simulink model "Y_Model_20_Loads"  (R2018b)
settings: Solver=VariableStepAuto  StartTime=0.0  StopTime=sim_t  RelTol=1e-3
values from neighbouring files (symbols this model uses):
  dt = 5e-5    (= 5e-05)    [Y_multi_sim_loads.m]
  L = ones(num_sims, num_loads) * L_max    [Y_multi_sim_loads.m]
  P = rand(num_sims, num_loads) * (P_max - P_min) + P_min    [Y_multi_sim_loads.m]
  R = ones(num_sims, num_loads) * R_max    [Y_multi_sim_loads.m]
libraries: powerlib x270, powerlib_meascontrol x56
(part 3 of 4)

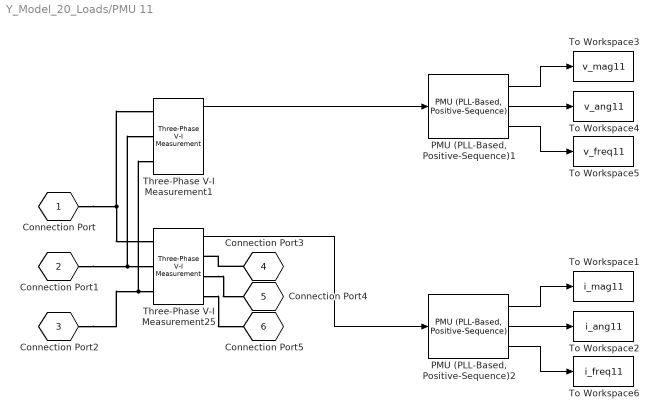
== system Y_Model_20_Loads/PMU 11 ==
  "PMU (PLL-Based, Positive-Sequence)1" : powerlib_meascontrol/Measurements/PMU (PLL-Based, Positive-Sequence)  nominalFrequency=50  samplingRate=64  reportingFactor=64
      settings: SourceProductName=Simscape Electrical  SourceProductBaseCode=PS
  "PMU (PLL-Based, Positive-Sequence)2" : powerlib_meascontrol/Measurements/PMU (PLL-Based, Positive-Sequence)  nominalFrequency=50  samplingRate=64  reportingFactor=64
      settings: SourceProductName=Simscape Electrical  SourceProductBaseCode=PS
  Three-Phase V-I Measurement1 : powerlib/Measurements/Three-Phase V-I Measurement  VoltageMeasurement=phase-to-ground  SetLabelV=off  LabelV=Vabc  Vpu=off  VpuLL=off  CurrentMeasurement=no  SetLabelI=off  LabelI=Iabc  Ipu=off  Pbase=100e6  Vbase=500e3  OutputType=Complex  PhasorSimulation=off  PSBequivalent=0
      settings: SourceProductName=Simscape Electrical
  Three-Phase V-I Measurement25 : powerlib/Measurements/Three-Phase V-I Measurement  VoltageMeasurement=no  SetLabelV=off  LabelV=Vabc  Vpu=off  VpuLL=off  CurrentMeasurement=yes  SetLabelI=off  LabelI=Iabc  Ipu=off  Pbase=100e6  Vbase=500e3  OutputType=Complex  PhasorSimulation=off  PSBequivalent=0
      settings: SourceProductName=Simscape Electrical
  To Workspace1 : ToWorkspace  VariableName=i_mag11  SampleTime=-1
  To Workspace2 : ToWorkspace  VariableName=i_ang11  SampleTime=-1
  To Workspace3 : ToWorkspace  VariableName=v_mag11  SampleTime=-1
  To Workspace4 : ToWorkspace  VariableName=v_ang11  SampleTime=-1
  To Workspace5 : ToWorkspace  VariableName=v_freq11  SampleTime=-1
  To Workspace6 : ToWorkspace  VariableName=i_freq11  SampleTime=-1
  Connection Port : PMIOPort  Tag=PMCPort  Side=Left
  Connection Port1 : PMIOPort  Tag=PMCPort  Port=2  Side=Left
  Connection Port2 : PMIOPort  Tag=PMCPort  Port=3  Side=Left
  Connection Port3 : PMIOPort  Tag=PMCPort  Port=4  Side=Right
  Connection Port4 : PMIOPort  Tag=PMCPort  Port=5  Side=Right
  Connection Port5 : PMIOPort  Tag=PMCPort  Port=6  Side=Right
  wires:
  "PMU (PLL-Based, Positive-Sequence)1"/3 -> To Workspace5/1
  "PMU (PLL-Based, Positive-Sequence)1"/2 -> To Workspace4/1
  "PMU (PLL-Based, Positive-Sequence)1"/1 -> To Workspace3/1
  "PMU (PLL-Based, Positive-Sequence)2"/3 -> To Workspace6/1
  "PMU (PLL-Based, Positive-Sequence)2"/1 -> To Workspace1/1
  "PMU (PLL-Based, Positive-Sequence)2"/2 -> To Workspace2/1
  Three-Phase V-I Measurement25/1 -> "PMU (PLL-Based, Positive-Sequence)2"/1
  Three-Phase V-I Measurement1/1 -> "PMU (PLL-Based, Positive-Sequence)1"/1
  connections:
  Three-Phase V-I Measurement25/LConn1 -- Connection Port/RConn1 -- Three-Phase V-I Measurement1/LConn1
  Connection Port1/RConn1 -- Three-Phase V-I Measurement1/LConn2 -- Three-Phase V-I Measurement25/LConn2
  Connection Port2/RConn1 -- Three-Phase V-I Measurement25/LConn3 -- Three-Phase V-I Measurement1/LConn3
  Connection Port3/RConn1 -- Three-Phase V-I Measurement25/RConn1
  Three-Phase V-I Measurement25/RConn2 -- Connection Port4/RConn1
  Three-Phase V-I Measurement25/RConn3 -- Connection Port5/RConn1

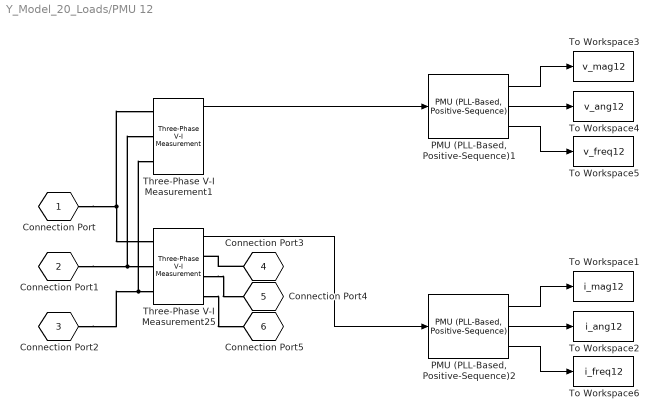
== system Y_Model_20_Loads/PMU 12 ==
  "PMU (PLL-Based, Positive-Sequence)1" : powerlib_meascontrol/Measurements/PMU (PLL-Based, Positive-Sequence)  nominalFrequency=50  samplingRate=64  reportingFactor=64
      settings: SourceProductName=Simscape Electrical  SourceProductBaseCode=PS
  "PMU (PLL-Based, Positive-Sequence)2" : powerlib_meascontrol/Measurements/PMU (PLL-Based, Positive-Sequence)  nominalFrequency=50  samplingRate=64  reportingFactor=64
      settings: SourceProductName=Simscape Electrical  SourceProductBaseCode=PS
  Three-Phase V-I Measurement1 : powerlib/Measurements/Three-Phase V-I Measurement  VoltageMeasurement=phase-to-ground  SetLabelV=off  LabelV=Vabc  Vpu=off  VpuLL=off  CurrentMeasurement=no  SetLabelI=off  LabelI=Iabc  Ipu=off  Pbase=100e6  Vbase=500e3  OutputType=Complex  PhasorSimulation=off  PSBequivalent=0
      settings: SourceProductName=Simscape Electrical
  Three-Phase V-I Measurement25 : powerlib/Measurements/Three-Phase V-I Measurement  VoltageMeasurement=no  SetLabelV=off  LabelV=Vabc  Vpu=off  VpuLL=off  CurrentMeasurement=yes  SetLabelI=off  LabelI=Iabc  Ipu=off  Pbase=100e6  Vbase=500e3  OutputType=Complex  PhasorSimulation=off  PSBequivalent=0
      settings: SourceProductName=Simscape Electrical
  To Workspace1 : ToWorkspace  VariableName=i_mag12  SampleTime=-1
  To Workspace2 : ToWorkspace  VariableName=i_ang12  SampleTime=-1
  To Workspace3 : ToWorkspace  VariableName=v_mag12  SampleTime=-1
  To Workspace4 : ToWorkspace  VariableName=v_ang12  SampleTime=-1
  To Workspace5 : ToWorkspace  VariableName=v_freq12  SampleTime=-1
  To Workspace6 : ToWorkspace  VariableName=i_freq12  SampleTime=-1
  Connection Port : PMIOPort  Tag=PMCPort  Side=Left
  Connection Port1 : PMIOPort  Tag=PMCPort  Port=2  Side=Left
  Connection Port2 : PMIOPort  Tag=PMCPort  Port=3  Side=Left
  Connection Port3 : PMIOPort  Tag=PMCPort  Port=4  Side=Right
  Connection Port4 : PMIOPort  Tag=PMCPort  Port=5  Side=Right
  Connection Port5 : PMIOPort  Tag=PMCPort  Port=6  Side=Right
  wires:
  "PMU (PLL-Based, Positive-Sequence)1"/3 -> To Workspace5/1
  "PMU (PLL-Based, Positive-Sequence)1"/2 -> To Workspace4/1
  "PMU (PLL-Based, Positive-Sequence)1"/1 -> To Workspace3/1
  "PMU (PLL-Based, Positive-Sequence)2"/3 -> To Workspace6/1
  "PMU (PLL-Based, Positive-Sequence)2"/1 -> To Workspace1/1
  "PMU (PLL-Based, Positive-Sequence)2"/2 -> To Workspace2/1
  Three-Phase V-I Measurement25/1 -> "PMU (PLL-Based, Positive-Sequence)2"/1
  Three-Phase V-I Measurement1/1 -> "PMU (PLL-Based, Positive-Sequence)1"/1
  connections:
  Three-Phase V-I Measurement25/LConn1 -- Connection Port/RConn1 -- Three-Phase V-I Measurement1/LConn1
  Connection Port1/RConn1 -- Three-Phase V-I Measurement1/LConn2 -- Three-Phase V-I Measurement25/LConn2
  Connection Port2/RConn1 -- Three-Phase V-I Measurement25/LConn3 -- Three-Phase V-I Measurement1/LConn3
  Connection Port3/RConn1 -- Three-Phase V-I Measurement25/RConn1
  Three-Phase V-I Measurement25/RConn2 -- Connection Port4/RConn1
  Three-Phase V-I Measurement25/RConn3 -- Connection Port5/RConn1

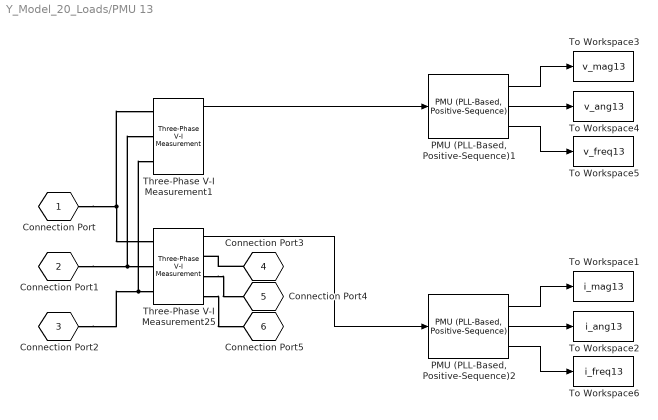
== system Y_Model_20_Loads/PMU 13 ==
  "PMU (PLL-Based, Positive-Sequence)1" : powerlib_meascontrol/Measurements/PMU (PLL-Based, Positive-Sequence)  nominalFrequency=50  samplingRate=64  reportingFactor=64
      settings: SourceProductName=Simscape Electrical  SourceProductBaseCode=PS
  "PMU (PLL-Based, Positive-Sequence)2" : powerlib_meascontrol/Measurements/PMU (PLL-Based, Positive-Sequence)  nominalFrequency=50  samplingRate=64  reportingFactor=64
      settings: SourceProductName=Simscape Electrical  SourceProductBaseCode=PS
  Three-Phase V-I Measurement1 : powerlib/Measurements/Three-Phase V-I Measurement  VoltageMeasurement=phase-to-ground  SetLabelV=off  LabelV=Vabc  Vpu=off  VpuLL=off  CurrentMeasurement=no  SetLabelI=off  LabelI=Iabc  Ipu=off  Pbase=100e6  Vbase=500e3  OutputType=Complex  PhasorSimulation=off  PSBequivalent=0
      settings: SourceProductName=Simscape Electrical
  Three-Phase V-I Measurement25 : powerlib/Measurements/Three-Phase V-I Measurement  VoltageMeasurement=no  SetLabelV=off  LabelV=Vabc  Vpu=off  VpuLL=off  CurrentMeasurement=yes  SetLabelI=off  LabelI=Iabc  Ipu=off  Pbase=100e6  Vbase=500e3  OutputType=Complex  PhasorSimulation=off  PSBequivalent=0
      settings: SourceProductName=Simscape Electrical
  To Workspace1 : ToWorkspace  VariableName=i_mag13  SampleTime=-1
  To Workspace2 : ToWorkspace  VariableName=i_ang13  SampleTime=-1
  To Workspace3 : ToWorkspace  VariableName=v_mag13  SampleTime=-1
  To Workspace4 : ToWorkspace  VariableName=v_ang13  SampleTime=-1
  To Workspace5 : ToWorkspace  VariableName=v_freq13  SampleTime=-1
  To Workspace6 : ToWorkspace  VariableName=i_freq13  SampleTime=-1
  Connection Port : PMIOPort  Tag=PMCPort  Side=Left
  Connection Port1 : PMIOPort  Tag=PMCPort  Port=2  Side=Left
  Connection Port2 : PMIOPort  Tag=PMCPort  Port=3  Side=Left
  Connection Port3 : PMIOPort  Tag=PMCPort  Port=4  Side=Right
  Connection Port4 : PMIOPort  Tag=PMCPort  Port=5  Side=Right
  Connection Port5 : PMIOPort  Tag=PMCPort  Port=6  Side=Right
  wires:
  "PMU (PLL-Based, Positive-Sequence)1"/3 -> To Workspace5/1
  "PMU (PLL-Based, Positive-Sequence)1"/2 -> To Workspace4/1
  "PMU (PLL-Based, Positive-Sequence)1"/1 -> To Workspace3/1
  "PMU (PLL-Based, Positive-Sequence)2"/3 -> To Workspace6/1
  "PMU (PLL-Based, Positive-Sequence)2"/1 -> To Workspace1/1
  "PMU (PLL-Based, Positive-Sequence)2"/2 -> To Workspace2/1
  Three-Phase V-I Measurement25/1 -> "PMU (PLL-Based, Positive-Sequence)2"/1
  Three-Phase V-I Measurement1/1 -> "PMU (PLL-Based, Positive-Sequence)1"/1
  connections:
  Three-Phase V-I Measurement25/LConn1 -- Connection Port/RConn1 -- Three-Phase V-I Measurement1/LConn1
  Connection Port1/RConn1 -- Three-Phase V-I Measurement1/LConn2 -- Three-Phase V-I Measurement25/LConn2
  Connection Port2/RConn1 -- Three-Phase V-I Measurement25/LConn3 -- Three-Phase V-I Measurement1/LConn3
  Connection Port3/RConn1 -- Three-Phase V-I Measurement25/RConn1
  Three-Phase V-I Measurement25/RConn2 -- Connection Port4/RConn1
  Three-Phase V-I Measurement25/RConn3 -- Connection Port5/RConn1

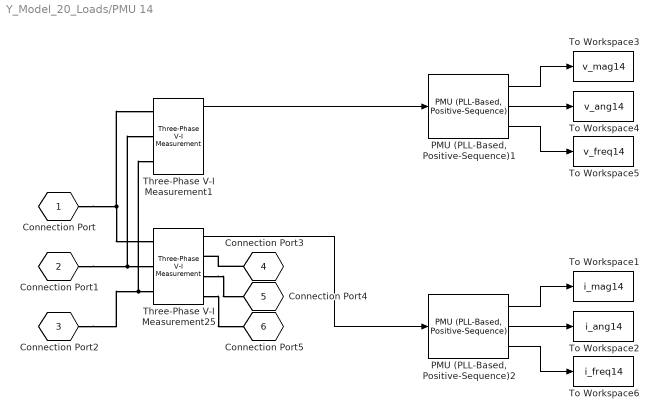
== system Y_Model_20_Loads/PMU 14 ==
  "PMU (PLL-Based, Positive-Sequence)1" : powerlib_meascontrol/Measurements/PMU (PLL-Based, Positive-Sequence)  nominalFrequency=50  samplingRate=64  reportingFactor=64
      settings: SourceProductName=Simscape Electrical  SourceProductBaseCode=PS
  "PMU (PLL-Based, Positive-Sequence)2" : powerlib_meascontrol/Measurements/PMU (PLL-Based, Positive-Sequence)  nominalFrequency=50  samplingRate=64  reportingFactor=64
      settings: SourceProductName=Simscape Electrical  SourceProductBaseCode=PS
  Three-Phase V-I Measurement1 : powerlib/Measurements/Three-Phase V-I Measurement  VoltageMeasurement=phase-to-ground  SetLabelV=off  LabelV=Vabc  Vpu=off  VpuLL=off  CurrentMeasurement=no  SetLabelI=off  LabelI=Iabc  Ipu=off  Pbase=100e6  Vbase=500e3  OutputType=Complex  PhasorSimulation=off  PSBequivalent=0
      settings: SourceProductName=Simscape Electrical
  Three-Phase V-I Measurement25 : powerlib/Measurements/Three-Phase V-I Measurement  VoltageMeasurement=no  SetLabelV=off  LabelV=Vabc  Vpu=off  VpuLL=off  CurrentMeasurement=yes  SetLabelI=off  LabelI=Iabc  Ipu=off  Pbase=100e6  Vbase=500e3  OutputType=Complex  PhasorSimulation=off  PSBequivalent=0
      settings: SourceProductName=Simscape Electrical
  To Workspace1 : ToWorkspace  VariableName=i_mag14  SampleTime=-1
  To Workspace2 : ToWorkspace  VariableName=i_ang14  SampleTime=-1
  To Workspace3 : ToWorkspace  VariableName=v_mag14  SampleTime=-1
  To Workspace4 : ToWorkspace  VariableName=v_ang14  SampleTime=-1
  To Workspace5 : ToWorkspace  VariableName=v_freq14  SampleTime=-1
  To Workspace6 : ToWorkspace  VariableName=i_freq14  SampleTime=-1
  Connection Port : PMIOPort  Tag=PMCPort  Side=Left
  Connection Port1 : PMIOPort  Tag=PMCPort  Port=2  Side=Left
  Connection Port2 : PMIOPort  Tag=PMCPort  Port=3  Side=Left
  Connection Port3 : PMIOPort  Tag=PMCPort  Port=4  Side=Right
  Connection Port4 : PMIOPort  Tag=PMCPort  Port=5  Side=Right
  Connection Port5 : PMIOPort  Tag=PMCPort  Port=6  Side=Right
  wires:
  "PMU (PLL-Based, Positive-Sequence)1"/3 -> To Workspace5/1
  "PMU (PLL-Based, Positive-Sequence)1"/2 -> To Workspace4/1
  "PMU (PLL-Based, Positive-Sequence)1"/1 -> To Workspace3/1
  "PMU (PLL-Based, Positive-Sequence)2"/3 -> To Workspace6/1
  "PMU (PLL-Based, Positive-Sequence)2"/1 -> To Workspace1/1
  "PMU (PLL-Based, Positive-Sequence)2"/2 -> To Workspace2/1
  Three-Phase V-I Measurement25/1 -> "PMU (PLL-Based, Positive-Sequence)2"/1
  Three-Phase V-I Measurement1/1 -> "PMU (PLL-Based, Positive-Sequence)1"/1
  connections:
  Three-Phase V-I Measurement25/LConn1 -- Connection Port/RConn1 -- Three-Phase V-I Measurement1/LConn1
  Connection Port1/RConn1 -- Three-Phase V-I Measurement1/LConn2 -- Three-Phase V-I Measurement25/LConn2
  Connection Port2/RConn1 -- Three-Phase V-I Measurement25/LConn3 -- Three-Phase V-I Measurement1/LConn3
  Connection Port3/RConn1 -- Three-Phase V-I Measurement25/RConn1
  Three-Phase V-I Measurement25/RConn2 -- Connection Port4/RConn1
  Three-Phase V-I Measurement25/RConn3 -- Connection Port5/RConn1

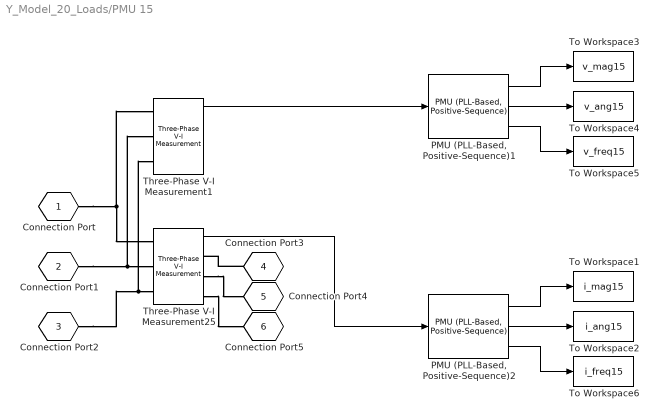
== system Y_Model_20_Loads/PMU 15 ==
  "PMU (PLL-Based, Positive-Sequence)1" : powerlib_meascontrol/Measurements/PMU (PLL-Based, Positive-Sequence)  nominalFrequency=50  samplingRate=64  reportingFactor=64
      settings: SourceProductName=Simscape Electrical  SourceProductBaseCode=PS
  "PMU (PLL-Based, Positive-Sequence)2" : powerlib_meascontrol/Measurements/PMU (PLL-Based, Positive-Sequence)  nominalFrequency=50  samplingRate=64  reportingFactor=64
      settings: SourceProductName=Simscape Electrical  SourceProductBaseCode=PS
  Three-Phase V-I Measurement1 : powerlib/Measurements/Three-Phase V-I Measurement  VoltageMeasurement=phase-to-ground  SetLabelV=off  LabelV=Vabc  Vpu=off  VpuLL=off  CurrentMeasurement=no  SetLabelI=off  LabelI=Iabc  Ipu=off  Pbase=100e6  Vbase=500e3  OutputType=Complex  PhasorSimulation=off  PSBequivalent=0
      settings: SourceProductName=Simscape Electrical
  Three-Phase V-I Measurement25 : powerlib/Measurements/Three-Phase V-I Measurement  VoltageMeasurement=no  SetLabelV=off  LabelV=Vabc  Vpu=off  VpuLL=off  CurrentMeasurement=yes  SetLabelI=off  LabelI=Iabc  Ipu=off  Pbase=100e6  Vbase=500e3  OutputType=Complex  PhasorSimulation=off  PSBequivalent=0
      settings: SourceProductName=Simscape Electrical
  To Workspace1 : ToWorkspace  VariableName=i_mag15  SampleTime=-1
  To Workspace2 : ToWorkspace  VariableName=i_ang15  SampleTime=-1
  To Workspace3 : ToWorkspace  VariableName=v_mag15  SampleTime=-1
  To Workspace4 : ToWorkspace  VariableName=v_ang15  SampleTime=-1
  To Workspace5 : ToWorkspace  VariableName=v_freq15  SampleTime=-1
  To Workspace6 : ToWorkspace  VariableName=i_freq15  SampleTime=-1
  Connection Port : PMIOPort  Tag=PMCPort  Side=Left
  Connection Port1 : PMIOPort  Tag=PMCPort  Port=2  Side=Left
  Connection Port2 : PMIOPort  Tag=PMCPort  Port=3  Side=Left
  Connection Port3 : PMIOPort  Tag=PMCPort  Port=4  Side=Right
  Connection Port4 : PMIOPort  Tag=PMCPort  Port=5  Side=Right
  Connection Port5 : PMIOPort  Tag=PMCPort  Port=6  Side=Right
  wires:
  "PMU (PLL-Based, Positive-Sequence)1"/3 -> To Workspace5/1
  "PMU (PLL-Based, Positive-Sequence)1"/2 -> To Workspace4/1
  "PMU (PLL-Based, Positive-Sequence)1"/1 -> To Workspace3/1
  "PMU (PLL-Based, Positive-Sequence)2"/3 -> To Workspace6/1
  "PMU (PLL-Based, Positive-Sequence)2"/1 -> To Workspace1/1
  "PMU (PLL-Based, Positive-Sequence)2"/2 -> To Workspace2/1
  Three-Phase V-I Measurement25/1 -> "PMU (PLL-Based, Positive-Sequence)2"/1
  Three-Phase V-I Measurement1/1 -> "PMU (PLL-Based, Positive-Sequence)1"/1
  connections:
  Three-Phase V-I Measurement25/LConn1 -- Connection Port/RConn1 -- Three-Phase V-I Measurement1/LConn1
  Connection Port1/RConn1 -- Three-Phase V-I Measurement1/LConn2 -- Three-Phase V-I Measurement25/LConn2
  Connection Port2/RConn1 -- Three-Phase V-I Measurement25/LConn3 -- Three-Phase V-I Measurement1/LConn3
  Connection Port3/RConn1 -- Three-Phase V-I Measurement25/RConn1
  Three-Phase V-I Measurement25/RConn2 -- Connection Port4/RConn1
  Three-Phase V-I Measurement25/RConn3 -- Connection Port5/RConn1

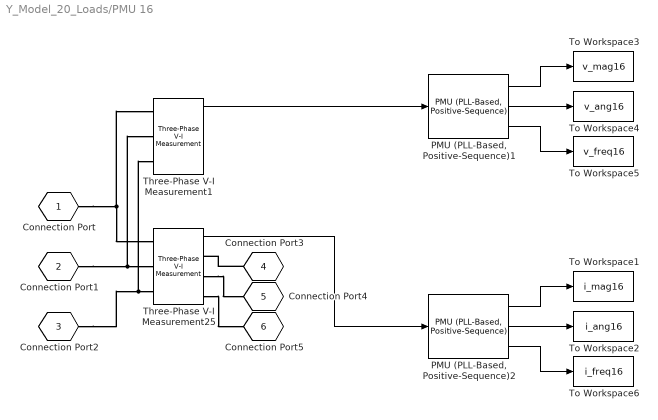
== system Y_Model_20_Loads/PMU 16 ==
  "PMU (PLL-Based, Positive-Sequence)1" : powerlib_meascontrol/Measurements/PMU (PLL-Based, Positive-Sequence)  nominalFrequency=50  samplingRate=64  reportingFactor=64
      settings: SourceProductName=Simscape Electrical  SourceProductBaseCode=PS
  "PMU (PLL-Based, Positive-Sequence)2" : powerlib_meascontrol/Measurements/PMU (PLL-Based, Positive-Sequence)  nominalFrequency=50  samplingRate=64  reportingFactor=64
      settings: SourceProductName=Simscape Electrical  SourceProductBaseCode=PS
  Three-Phase V-I Measurement1 : powerlib/Measurements/Three-Phase V-I Measurement  VoltageMeasurement=phase-to-ground  SetLabelV=off  LabelV=Vabc  Vpu=off  VpuLL=off  CurrentMeasurement=no  SetLabelI=off  LabelI=Iabc  Ipu=off  Pbase=100e6  Vbase=500e3  OutputType=Complex  PhasorSimulation=off  PSBequivalent=0
      settings: SourceProductName=Simscape Electrical
  Three-Phase V-I Measurement25 : powerlib/Measurements/Three-Phase V-I Measurement  VoltageMeasurement=no  SetLabelV=off  LabelV=Vabc  Vpu=off  VpuLL=off  CurrentMeasurement=yes  SetLabelI=off  LabelI=Iabc  Ipu=off  Pbase=100e6  Vbase=500e3  OutputType=Complex  PhasorSimulation=off  PSBequivalent=0
      settings: SourceProductName=Simscape Electrical
  To Workspace1 : ToWorkspace  VariableName=i_mag16  SampleTime=-1
  To Workspace2 : ToWorkspace  VariableName=i_ang16  SampleTime=-1
  To Workspace3 : ToWorkspace  VariableName=v_mag16  SampleTime=-1
  To Workspace4 : ToWorkspace  VariableName=v_ang16  SampleTime=-1
  To Workspace5 : ToWorkspace  VariableName=v_freq16  SampleTime=-1
  To Workspace6 : ToWorkspace  VariableName=i_freq16  SampleTime=-1
  Connection Port : PMIOPort  Tag=PMCPort  Side=Left
  Connection Port1 : PMIOPort  Tag=PMCPort  Port=2  Side=Left
  Connection Port2 : PMIOPort  Tag=PMCPort  Port=3  Side=Left
  Connection Port3 : PMIOPort  Tag=PMCPort  Port=4  Side=Right
  Connection Port4 : PMIOPort  Tag=PMCPort  Port=5  Side=Right
  Connection Port5 : PMIOPort  Tag=PMCPort  Port=6  Side=Right
  wires:
  "PMU (PLL-Based, Positive-Sequence)1"/3 -> To Workspace5/1
  "PMU (PLL-Based, Positive-Sequence)1"/2 -> To Workspace4/1
  "PMU (PLL-Based, Positive-Sequence)1"/1 -> To Workspace3/1
  "PMU (PLL-Based, Positive-Sequence)2"/3 -> To Workspace6/1
  "PMU (PLL-Based, Positive-Sequence)2"/1 -> To Workspace1/1
  "PMU (PLL-Based, Positive-Sequence)2"/2 -> To Workspace2/1
  Three-Phase V-I Measurement25/1 -> "PMU (PLL-Based, Positive-Sequence)2"/1
  Three-Phase V-I Measurement1/1 -> "PMU (PLL-Based, Positive-Sequence)1"/1
  connections:
  Three-Phase V-I Measurement25/LConn1 -- Connection Port/RConn1 -- Three-Phase V-I Measurement1/LConn1
  Connection Port1/RConn1 -- Three-Phase V-I Measurement1/LConn2 -- Three-Phase V-I Measurement25/LConn2
  Connection Port2/RConn1 -- Three-Phase V-I Measurement25/LConn3 -- Three-Phase V-I Measurement1/LConn3
  Connection Port3/RConn1 -- Three-Phase V-I Measurement25/RConn1
  Three-Phase V-I Measurement25/RConn2 -- Connection Port4/RConn1
  Three-Phase V-I Measurement25/RConn3 -- Connection Port5/RConn1

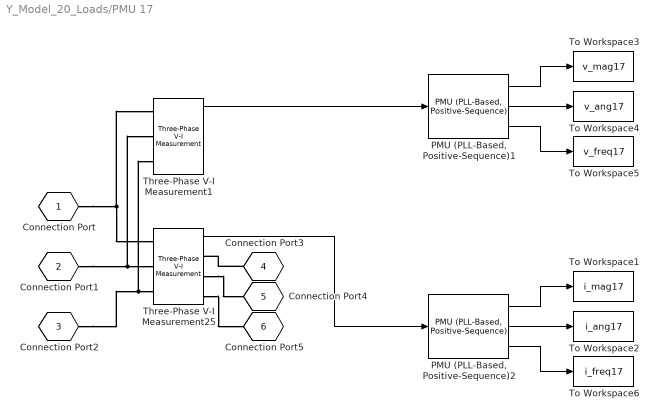
== system Y_Model_20_Loads/PMU 17 ==
  "PMU (PLL-Based, Positive-Sequence)1" : powerlib_meascontrol/Measurements/PMU (PLL-Based, Positive-Sequence)  nominalFrequency=50  samplingRate=64  reportingFactor=64
      settings: SourceProductName=Simscape Electrical  SourceProductBaseCode=PS
  "PMU (PLL-Based, Positive-Sequence)2" : powerlib_meascontrol/Measurements/PMU (PLL-Based, Positive-Sequence)  nominalFrequency=50  samplingRate=64  reportingFactor=64
      settings: SourceProductName=Simscape Electrical  SourceProductBaseCode=PS
  Three-Phase V-I Measurement1 : powerlib/Measurements/Three-Phase V-I Measurement  VoltageMeasurement=phase-to-ground  SetLabelV=off  LabelV=Vabc  Vpu=off  VpuLL=off  CurrentMeasurement=no  SetLabelI=off  LabelI=Iabc  Ipu=off  Pbase=100e6  Vbase=500e3  OutputType=Complex  PhasorSimulation=off  PSBequivalent=0
      settings: SourceProductName=Simscape Electrical
  Three-Phase V-I Measurement25 : powerlib/Measurements/Three-Phase V-I Measurement  VoltageMeasurement=no  SetLabelV=off  LabelV=Vabc  Vpu=off  VpuLL=off  CurrentMeasurement=yes  SetLabelI=off  LabelI=Iabc  Ipu=off  Pbase=100e6  Vbase=500e3  OutputType=Complex  PhasorSimulation=off  PSBequivalent=0
      settings: SourceProductName=Simscape Electrical
  To Workspace1 : ToWorkspace  VariableName=i_mag17  SampleTime=-1
  To Workspace2 : ToWorkspace  VariableName=i_ang17  SampleTime=-1
  To Workspace3 : ToWorkspace  VariableName=v_mag17  SampleTime=-1
  To Workspace4 : ToWorkspace  VariableName=v_ang17  SampleTime=-1
  To Workspace5 : ToWorkspace  VariableName=v_freq17  SampleTime=-1
  To Workspace6 : ToWorkspace  VariableName=i_freq17  SampleTime=-1
  Connection Port : PMIOPort  Tag=PMCPort  Side=Left
  Connection Port1 : PMIOPort  Tag=PMCPort  Port=2  Side=Left
  Connection Port2 : PMIOPort  Tag=PMCPort  Port=3  Side=Left
  Connection Port3 : PMIOPort  Tag=PMCPort  Port=4  Side=Right
  Connection Port4 : PMIOPort  Tag=PMCPort  Port=5  Side=Right
  Connection Port5 : PMIOPort  Tag=PMCPort  Port=6  Side=Right
  wires:
  "PMU (PLL-Based, Positive-Sequence)1"/3 -> To Workspace5/1
  "PMU (PLL-Based, Positive-Sequence)1"/2 -> To Workspace4/1
  "PMU (PLL-Based, Positive-Sequence)1"/1 -> To Workspace3/1
  "PMU (PLL-Based, Positive-Sequence)2"/3 -> To Workspace6/1
  "PMU (PLL-Based, Positive-Sequence)2"/1 -> To Workspace1/1
  "PMU (PLL-Based, Positive-Sequence)2"/2 -> To Workspace2/1
  Three-Phase V-I Measurement25/1 -> "PMU (PLL-Based, Positive-Sequence)2"/1
  Three-Phase V-I Measurement1/1 -> "PMU (PLL-Based, Positive-Sequence)1"/1
  connections:
  Three-Phase V-I Measurement25/LConn1 -- Connection Port/RConn1 -- Three-Phase V-I Measurement1/LConn1
  Connection Port1/RConn1 -- Three-Phase V-I Measurement1/LConn2 -- Three-Phase V-I Measurement25/LConn2
  Connection Port2/RConn1 -- Three-Phase V-I Measurement25/LConn3 -- Three-Phase V-I Measurement1/LConn3
  Connection Port3/RConn1 -- Three-Phase V-I Measurement25/RConn1
  Three-Phase V-I Measurement25/RConn2 -- Connection Port4/RConn1
  Three-Phase V-I Measurement25/RConn3 -- Connection Port5/RConn1

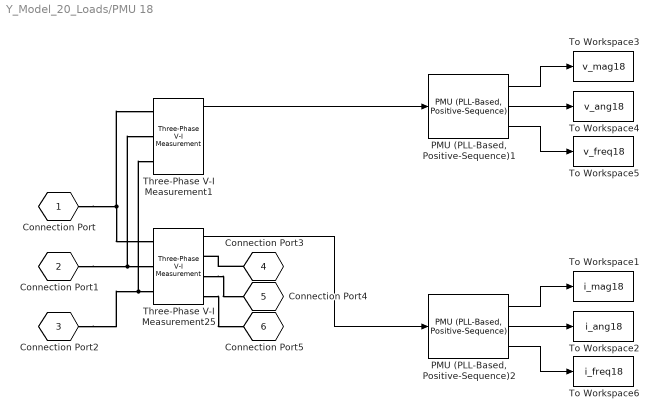
== system Y_Model_20_Loads/PMU 18 ==
  "PMU (PLL-Based, Positive-Sequence)1" : powerlib_meascontrol/Measurements/PMU (PLL-Based, Positive-Sequence)  nominalFrequency=50  samplingRate=64  reportingFactor=64
      settings: SourceProductName=Simscape Electrical  SourceProductBaseCode=PS
  "PMU (PLL-Based, Positive-Sequence)2" : powerlib_meascontrol/Measurements/PMU (PLL-Based, Positive-Sequence)  nominalFrequency=50  samplingRate=64  reportingFactor=64
      settings: SourceProductName=Simscape Electrical  SourceProductBaseCode=PS
  Three-Phase V-I Measurement1 : powerlib/Measurements/Three-Phase V-I Measurement  VoltageMeasurement=phase-to-ground  SetLabelV=off  LabelV=Vabc  Vpu=off  VpuLL=off  CurrentMeasurement=no  SetLabelI=off  LabelI=Iabc  Ipu=off  Pbase=100e6  Vbase=500e3  OutputType=Complex  PhasorSimulation=off  PSBequivalent=0
      settings: SourceProductName=Simscape Electrical
  Three-Phase V-I Measurement25 : powerlib/Measurements/Three-Phase V-I Measurement  VoltageMeasurement=no  SetLabelV=off  LabelV=Vabc  Vpu=off  VpuLL=off  CurrentMeasurement=yes  SetLabelI=off  LabelI=Iabc  Ipu=off  Pbase=100e6  Vbase=500e3  OutputType=Complex  PhasorSimulation=off  PSBequivalent=0
      settings: SourceProductName=Simscape Electrical
  To Workspace1 : ToWorkspace  VariableName=i_mag18  SampleTime=-1
  To Workspace2 : ToWorkspace  VariableName=i_ang18  SampleTime=-1
  To Workspace3 : ToWorkspace  VariableName=v_mag18  SampleTime=-1
  To Workspace4 : ToWorkspace  VariableName=v_ang18  SampleTime=-1
  To Workspace5 : ToWorkspace  VariableName=v_freq18  SampleTime=-1
  To Workspace6 : ToWorkspace  VariableName=i_freq18  SampleTime=-1
  Connection Port : PMIOPort  Tag=PMCPort  Side=Left
  Connection Port1 : PMIOPort  Tag=PMCPort  Port=2  Side=Left
  Connection Port2 : PMIOPort  Tag=PMCPort  Port=3  Side=Left
  Connection Port3 : PMIOPort  Tag=PMCPort  Port=4  Side=Right
  Connection Port4 : PMIOPort  Tag=PMCPort  Port=5  Side=Right
  Connection Port5 : PMIOPort  Tag=PMCPort  Port=6  Side=Right
  wires:
  "PMU (PLL-Based, Positive-Sequence)1"/3 -> To Workspace5/1
  "PMU (PLL-Based, Positive-Sequence)1"/2 -> To Workspace4/1
  "PMU (PLL-Based, Positive-Sequence)1"/1 -> To Workspace3/1
  "PMU (PLL-Based, Positive-Sequence)2"/3 -> To Workspace6/1
  "PMU (PLL-Based, Positive-Sequence)2"/1 -> To Workspace1/1
  "PMU (PLL-Based, Positive-Sequence)2"/2 -> To Workspace2/1
  Three-Phase V-I Measurement25/1 -> "PMU (PLL-Based, Positive-Sequence)2"/1
  Three-Phase V-I Measurement1/1 -> "PMU (PLL-Based, Positive-Sequence)1"/1
  connections:
  Three-Phase V-I Measurement25/LConn1 -- Connection Port/RConn1 -- Three-Phase V-I Measurement1/LConn1
  Connection Port1/RConn1 -- Three-Phase V-I Measurement1/LConn2 -- Three-Phase V-I Measurement25/LConn2
  Connection Port2/RConn1 -- Three-Phase V-I Measurement25/LConn3 -- Three-Phase V-I Measurement1/LConn3
  Connection Port3/RConn1 -- Three-Phase V-I Measurement25/RConn1
  Three-Phase V-I Measurement25/RConn2 -- Connection Port4/RConn1
  Three-Phase V-I Measurement25/RConn3 -- Connection Port5/RConn1

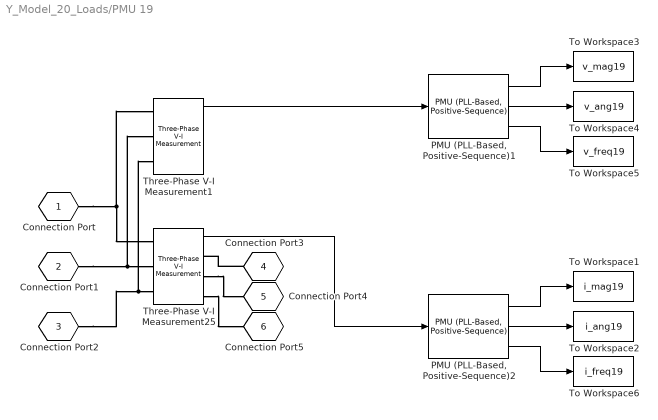
== system Y_Model_20_Loads/PMU 19 ==
  "PMU (PLL-Based, Positive-Sequence)1" : powerlib_meascontrol/Measurements/PMU (PLL-Based, Positive-Sequence)  nominalFrequency=50  samplingRate=64  reportingFactor=64
      settings: SourceProductName=Simscape Electrical  SourceProductBaseCode=PS
  "PMU (PLL-Based, Positive-Sequence)2" : powerlib_meascontrol/Measurements/PMU (PLL-Based, Positive-Sequence)  nominalFrequency=50  samplingRate=64  reportingFactor=64
      settings: SourceProductName=Simscape Electrical  SourceProductBaseCode=PS
  Three-Phase V-I Measurement1 : powerlib/Measurements/Three-Phase V-I Measurement  VoltageMeasurement=phase-to-ground  SetLabelV=off  LabelV=Vabc  Vpu=off  VpuLL=off  CurrentMeasurement=no  SetLabelI=off  LabelI=Iabc  Ipu=off  Pbase=100e6  Vbase=500e3  OutputType=Complex  PhasorSimulation=off  PSBequivalent=0
      settings: SourceProductName=Simscape Electrical
  Three-Phase V-I Measurement25 : powerlib/Measurements/Three-Phase V-I Measurement  VoltageMeasurement=no  SetLabelV=off  LabelV=Vabc  Vpu=off  VpuLL=off  CurrentMeasurement=yes  SetLabelI=off  LabelI=Iabc  Ipu=off  Pbase=100e6  Vbase=500e3  OutputType=Complex  PhasorSimulation=off  PSBequivalent=0
      settings: SourceProductName=Simscape Electrical
  To Workspace1 : ToWorkspace  VariableName=i_mag19  SampleTime=-1
  To Workspace2 : ToWorkspace  VariableName=i_ang19  SampleTime=-1
  To Workspace3 : ToWorkspace  VariableName=v_mag19  SampleTime=-1
  To Workspace4 : ToWorkspace  VariableName=v_ang19  SampleTime=-1
  To Workspace5 : ToWorkspace  VariableName=v_freq19  SampleTime=-1
  To Workspace6 : ToWorkspace  VariableName=i_freq19  SampleTime=-1
  Connection Port : PMIOPort  Tag=PMCPort  Side=Left
  Connection Port1 : PMIOPort  Tag=PMCPort  Port=2  Side=Left
  Connection Port2 : PMIOPort  Tag=PMCPort  Port=3  Side=Left
  Connection Port3 : PMIOPort  Tag=PMCPort  Port=4  Side=Right
  Connection Port4 : PMIOPort  Tag=PMCPort  Port=5  Side=Right
  Connection Port5 : PMIOPort  Tag=PMCPort  Port=6  Side=Right
  wires:
  "PMU (PLL-Based, Positive-Sequence)1"/3 -> To Workspace5/1
  "PMU (PLL-Based, Positive-Sequence)1"/2 -> To Workspace4/1
  "PMU (PLL-Based, Positive-Sequence)1"/1 -> To Workspace3/1
  "PMU (PLL-Based, Positive-Sequence)2"/3 -> To Workspace6/1
  "PMU (PLL-Based, Positive-Sequence)2"/1 -> To Workspace1/1
  "PMU (PLL-Based, Positive-Sequence)2"/2 -> To Workspace2/1
  Three-Phase V-I Measurement25/1 -> "PMU (PLL-Based, Positive-Sequence)2"/1
  Three-Phase V-I Measurement1/1 -> "PMU (PLL-Based, Positive-Sequence)1"/1
  connections:
  Three-Phase V-I Measurement25/LConn1 -- Connection Port/RConn1 -- Three-Phase V-I Measurement1/LConn1
  Connection Port1/RConn1 -- Three-Phase V-I Measurement1/LConn2 -- Three-Phase V-I Measurement25/LConn2
  Connection Port2/RConn1 -- Three-Phase V-I Measurement25/LConn3 -- Three-Phase V-I Measurement1/LConn3
  Connection Port3/RConn1 -- Three-Phase V-I Measurement25/RConn1
  Three-Phase V-I Measurement25/RConn2 -- Connection Port4/RConn1
  Three-Phase V-I Measurement25/RConn3 -- Connection Port5/RConn1

== system Y_Model_20_Loads/PMU 2 ==
  "PMU (PLL-Based, Positive-Sequence)1" : powerlib_meascontrol/Measurements/PMU (PLL-Based, Positive-Sequence)  nominalFrequency=50  samplingRate=64  reportingFactor=64
      settings: SourceProductName=Simscape Electrical  SourceProductBaseCode=PS
  "PMU (PLL-Based, Positive-Sequence)2" : powerlib_meascontrol/Measurements/PMU (PLL-Based, Positive-Sequence)  nominalFrequency=50  samplingRate=64  reportingFactor=64
      settings: SourceProductName=Simscape Electrical  SourceProductBaseCode=PS
  Three-Phase V-I Measurement1 : powerlib/Measurements/Three-Phase V-I Measurement  VoltageMeasurement=phase-to-ground  SetLabelV=off  LabelV=Vabc  Vpu=off  VpuLL=off  CurrentMeasurement=no  SetLabelI=off  LabelI=Iabc  Ipu=off  Pbase=100e6  Vbase=500e3  OutputType=Complex  PhasorSimulation=off  PSBequivalent=0
      settings: SourceProductName=Simscape Electrical
  Three-Phase V-I Measurement25 : powerlib/Measurements/Three-Phase V-I Measurement  VoltageMeasurement=no  SetLabelV=off  LabelV=Vabc  Vpu=off  VpuLL=off  CurrentMeasurement=yes  SetLabelI=off  LabelI=Iabc  Ipu=off  Pbase=100e6  Vbase=500e3  OutputType=Complex  PhasorSimulation=off  PSBequivalent=0
      settings: SourceProductName=Simscape Electrical
  To Workspace1 : ToWorkspace  VariableName=i_mag2  SampleTime=-1
  To Workspace2 : ToWorkspace  VariableName=i_ang2  SampleTime=-1
  To Workspace3 : ToWorkspace  VariableName=v_mag2  SampleTime=-1
  To Workspace4 : ToWorkspace  VariableName=v_ang2  SampleTime=-1
  To Workspace5 : ToWorkspace  VariableName=v_freq2  SampleTime=-1
  To Workspace6 : ToWorkspace  VariableName=i_freq2  SampleTime=-1
  Connection Port : PMIOPort  Tag=PMCPort  Side=Left
  Connection Port1 : PMIOPort  Tag=PMCPort  Port=2  Side=Left
  Connection Port2 : PMIOPort  Tag=PMCPort  Port=3  Side=Left
  Connection Port3 : PMIOPort  Tag=PMCPort  Port=4  Side=Right
  Connection Port4 : PMIOPort  Tag=PMCPort  Port=5  Side=Right
  Connection Port5 : PMIOPort  Tag=PMCPort  Port=6  Side=Right
  wires:
  "PMU (PLL-Based, Positive-Sequence)1"/3 -> To Workspace5/1
  "PMU (PLL-Based, Positive-Sequence)1"/2 -> To Workspace4/1
  "PMU (PLL-Based, Positive-Sequence)1"/1 -> To Workspace3/1
  "PMU (PLL-Based, Positive-Sequence)2"/3 -> To Workspace6/1
  "PMU (PLL-Based, Positive-Sequence)2"/1 -> To Workspace1/1
  "PMU (PLL-Based, Positive-Sequence)2"/2 -> To Workspace2/1
  Three-Phase V-I Measurement25/1 -> "PMU (PLL-Based, Positive-Sequence)2"/1
  Three-Phase V-I Measurement1/1 -> "PMU (PLL-Based, Positive-Sequence)1"/1
  connections:
  Three-Phase V-I Measurement25/LConn1 -- Connection Port/RConn1 -- Three-Phase V-I Measurement1/LConn1
  Connection Port1/RConn1 -- Three-Phase V-I Measurement1/LConn2 -- Three-Phase V-I Measurement25/LConn2
  Connection Port2/RConn1 -- Three-Phase V-I Measurement25/LConn3 -- Three-Phase V-I Measurement1/LConn3
  Connection Port3/RConn1 -- Three-Phase V-I Measurement25/RConn1
  Three-Phase V-I Measurement25/RConn2 -- Connection Port4/RConn1
  Three-Phase V-I Measurement25/RConn3 -- Connection Port5/RConn1

== system Y_Model_20_Loads/PMU 20 ==
  "PMU (PLL-Based, Positive-Sequence)1" : powerlib_meascontrol/Measurements/PMU (PLL-Based, Positive-Sequence)  nominalFrequency=50  samplingRate=64  reportingFactor=64
      settings: SourceProductName=Simscape Electrical  SourceProductBaseCode=PS
  "PMU (PLL-Based, Positive-Sequence)2" : powerlib_meascontrol/Measurements/PMU (PLL-Based, Positive-Sequence)  nominalFrequency=50  samplingRate=64  reportingFactor=64
      settings: SourceProductName=Simscape Electrical  SourceProductBaseCode=PS
  Three-Phase V-I Measurement1 : powerlib/Measurements/Three-Phase V-I Measurement  VoltageMeasurement=phase-to-ground  SetLabelV=off  LabelV=Vabc  Vpu=off  VpuLL=off  CurrentMeasurement=no  SetLabelI=off  LabelI=Iabc  Ipu=off  Pbase=100e6  Vbase=500e3  OutputType=Complex  PhasorSimulation=off  PSBequivalent=0
      settings: SourceProductName=Simscape Electrical
  Three-Phase V-I Measurement25 : powerlib/Measurements/Three-Phase V-I Measurement  VoltageMeasurement=no  SetLabelV=off  LabelV=Vabc  Vpu=off  VpuLL=off  CurrentMeasurement=yes  SetLabelI=off  LabelI=Iabc  Ipu=off  Pbase=100e6  Vbase=500e3  OutputType=Complex  PhasorSimulation=off  PSBequivalent=0
      settings: SourceProductName=Simscape Electrical
  To Workspace1 : ToWorkspace  VariableName=i_mag20  SampleTime=-1
  To Workspace2 : ToWorkspace  VariableName=i_ang20  SampleTime=-1
  To Workspace3 : ToWorkspace  VariableName=v_mag20  SampleTime=-1
  To Workspace4 : ToWorkspace  VariableName=v_ang20  SampleTime=-1
  To Workspace5 : ToWorkspace  VariableName=v_freq20  SampleTime=-1
  To Workspace6 : ToWorkspace  VariableName=i_freq20  SampleTime=-1
  Connection Port : PMIOPort  Tag=PMCPort  Side=Left
  Connection Port1 : PMIOPort  Tag=PMCPort  Port=2  Side=Left
  Connection Port2 : PMIOPort  Tag=PMCPort  Port=3  Side=Left
  Connection Port3 : PMIOPort  Tag=PMCPort  Port=4  Side=Right
  Connection Port4 : PMIOPort  Tag=PMCPort  Port=5  Side=Right
  Connection Port5 : PMIOPort  Tag=PMCPort  Port=6  Side=Right
  wires:
  "PMU (PLL-Based, Positive-Sequence)1"/3 -> To Workspace5/1
  "PMU (PLL-Based, Positive-Sequence)1"/2 -> To Workspace4/1
  "PMU (PLL-Based, Positive-Sequence)1"/1 -> To Workspace3/1
  "PMU (PLL-Based, Positive-Sequence)2"/3 -> To Workspace6/1
  "PMU (PLL-Based, Positive-Sequence)2"/1 -> To Workspace1/1
  "PMU (PLL-Based, Positive-Sequence)2"/2 -> To Workspace2/1
  Three-Phase V-I Measurement25/1 -> "PMU (PLL-Based, Positive-Sequence)2"/1
  Three-Phase V-I Measurement1/1 -> "PMU (PLL-Based, Positive-Sequence)1"/1
  connections:
  Three-Phase V-I Measurement25/LConn1 -- Connection Port/RConn1 -- Three-Phase V-I Measurement1/LConn1
  Connection Port1/RConn1 -- Three-Phase V-I Measurement1/LConn2 -- Three-Phase V-I Measurement25/LConn2
  Connection Port2/RConn1 -- Three-Phase V-I Measurement25/LConn3 -- Three-Phase V-I Measurement1/LConn3
  Connection Port3/RConn1 -- Three-Phase V-I Measurement25/RConn1
  Three-Phase V-I Measurement25/RConn2 -- Connection Port4/RConn1
  Three-Phase V-I Measurement25/RConn3 -- Connection Port5/RConn1

== system Y_Model_20_Loads/PMU 21 ==
  "PMU (PLL-Based, Positive-Sequence)1" : powerlib_meascontrol/Measurements/PMU (PLL-Based, Positive-Sequence)  nominalFrequency=50  samplingRate=64  reportingFactor=64
      settings: SourceProductName=Simscape Electrical  SourceProductBaseCode=PS
  "PMU (PLL-Based, Positive-Sequence)2" : powerlib_meascontrol/Measurements/PMU (PLL-Based, Positive-Sequence)  nominalFrequency=50  samplingRate=64  reportingFactor=64
      settings: SourceProductName=Simscape Electrical  SourceProductBaseCode=PS
  Three-Phase V-I Measurement1 : powerlib/Measurements/Three-Phase V-I Measurement  VoltageMeasurement=phase-to-ground  SetLabelV=off  LabelV=Vabc  Vpu=off  VpuLL=off  CurrentMeasurement=no  SetLabelI=off  LabelI=Iabc  Ipu=off  Pbase=100e6  Vbase=500e3  OutputType=Complex  PhasorSimulation=off  PSBequivalent=0
      settings: SourceProductName=Simscape Electrical
  Three-Phase V-I Measurement25 : powerlib/Measurements/Three-Phase V-I Measurement  VoltageMeasurement=no  SetLabelV=off  LabelV=Vabc  Vpu=off  VpuLL=off  CurrentMeasurement=yes  SetLabelI=off  LabelI=Iabc  Ipu=off  Pbase=100e6  Vbase=500e3  OutputType=Complex  PhasorSimulation=off  PSBequivalent=0
      settings: SourceProductName=Simscape Electrical
  To Workspace1 : ToWorkspace  VariableName=i_mag21  SampleTime=-1
  To Workspace2 : ToWorkspace  VariableName=i_ang21  SampleTime=-1
  To Workspace3 : ToWorkspace  VariableName=v_mag21  SampleTime=-1
  To Workspace4 : ToWorkspace  VariableName=v_ang21  SampleTime=-1
  To Workspace5 : ToWorkspace  VariableName=v_freq21  SampleTime=-1
  To Workspace6 : ToWorkspace  VariableName=i_freq21  SampleTime=-1
  Connection Port : PMIOPort  Tag=PMCPort  Side=Left
  Connection Port1 : PMIOPort  Tag=PMCPort  Port=2  Side=Left
  Connection Port2 : PMIOPort  Tag=PMCPort  Port=3  Side=Left
  Connection Port3 : PMIOPort  Tag=PMCPort  Port=4  Side=Right
  Connection Port4 : PMIOPort  Tag=PMCPort  Port=5  Side=Right
  Connection Port5 : PMIOPort  Tag=PMCPort  Port=6  Side=Right
  wires:
  "PMU (PLL-Based, Positive-Sequence)1"/3 -> To Workspace5/1
  "PMU (PLL-Based, Positive-Sequence)1"/2 -> To Workspace4/1
  "PMU (PLL-Based, Positive-Sequence)1"/1 -> To Workspace3/1
  "PMU (PLL-Based, Positive-Sequence)2"/3 -> To Workspace6/1
  "PMU (PLL-Based, Positive-Sequence)2"/1 -> To Workspace1/1
  "PMU (PLL-Based, Positive-Sequence)2"/2 -> To Workspace2/1
  Three-Phase V-I Measurement25/1 -> "PMU (PLL-Based, Positive-Sequence)2"/1
  Three-Phase V-I Measurement1/1 -> "PMU (PLL-Based, Positive-Sequence)1"/1
  connections:
  Three-Phase V-I Measurement25/LConn1 -- Connection Port/RConn1 -- Three-Phase V-I Measurement1/LConn1
  Connection Port1/RConn1 -- Three-Phase V-I Measurement1/LConn2 -- Three-Phase V-I Measurement25/LConn2
  Connection Port2/RConn1 -- Three-Phase V-I Measurement25/LConn3 -- Three-Phase V-I Measurement1/LConn3
  Connection Port3/RConn1 -- Three-Phase V-I Measurement25/RConn1
  Three-Phase V-I Measurement25/RConn2 -- Connection Port4/RConn1
  Three-Phase V-I Measurement25/RConn3 -- Connection Port5/RConn1

== system Y_Model_20_Loads/PMU 3 ==
  "PMU (PLL-Based, Positive-Sequence)1" : powerlib_meascontrol/Measurements/PMU (PLL-Based, Positive-Sequence)  nominalFrequency=50  samplingRate=64  reportingFactor=64
      settings: SourceProductName=Simscape Electrical  SourceProductBaseCode=PS
  "PMU (PLL-Based, Positive-Sequence)2" : powerlib_meascontrol/Measurements/PMU (PLL-Based, Positive-Sequence)  nominalFrequency=50  samplingRate=64  reportingFactor=64
      settings: SourceProductName=Simscape Electrical  SourceProductBaseCode=PS
  Three-Phase V-I Measurement1 : powerlib/Measurements/Three-Phase V-I Measurement  VoltageMeasurement=phase-to-ground  SetLabelV=off  LabelV=Vabc  Vpu=off  VpuLL=off  CurrentMeasurement=no  SetLabelI=off  LabelI=Iabc  Ipu=off  Pbase=100e6  Vbase=500e3  OutputType=Complex  PhasorSimulation=off  PSBequivalent=0
      settings: SourceProductName=Simscape Electrical
  Three-Phase V-I Measurement25 : powerlib/Measurements/Three-Phase V-I Measurement  VoltageMeasurement=no  SetLabelV=off  LabelV=Vabc  Vpu=off  VpuLL=off  CurrentMeasurement=yes  SetLabelI=off  LabelI=Iabc  Ipu=off  Pbase=100e6  Vbase=500e3  OutputType=Complex  PhasorSimulation=off  PSBequivalent=0
      settings: SourceProductName=Simscape Electrical
  To Workspace1 : ToWorkspace  VariableName=i_mag3  SampleTime=-1
  To Workspace2 : ToWorkspace  VariableName=i_ang3  SampleTime=-1
  To Workspace3 : ToWorkspace  VariableName=v_mag3  SampleTime=-1
  To Workspace4 : ToWorkspace  VariableName=v_ang3  SampleTime=-1
  To Workspace5 : ToWorkspace  VariableName=v_freq3  SampleTime=-1
  To Workspace6 : ToWorkspace  VariableName=i_freq3  SampleTime=-1
  Connection Port : PMIOPort  Tag=PMCPort  Side=Left
  Connection Port1 : PMIOPort  Tag=PMCPort  Port=2  Side=Left
  Connection Port2 : PMIOPort  Tag=PMCPort  Port=3  Side=Left
  Connection Port3 : PMIOPort  Tag=PMCPort  Port=4  Side=Right
  Connection Port4 : PMIOPort  Tag=PMCPort  Port=5  Side=Right
  Connection Port5 : PMIOPort  Tag=PMCPort  Port=6  Side=Right
  wires:
  "PMU (PLL-Based, Positive-Sequence)1"/3 -> To Workspace5/1
  "PMU (PLL-Based, Positive-Sequence)1"/2 -> To Workspace4/1
  "PMU (PLL-Based, Positive-Sequence)1"/1 -> To Workspace3/1
  "PMU (PLL-Based, Positive-Sequence)2"/3 -> To Workspace6/1
  "PMU (PLL-Based, Positive-Sequence)2"/1 -> To Workspace1/1
  "PMU (PLL-Based, Positive-Sequence)2"/2 -> To Workspace2/1
  Three-Phase V-I Measurement25/1 -> "PMU (PLL-Based, Positive-Sequence)2"/1
  Three-Phase V-I Measurement1/1 -> "PMU (PLL-Based, Positive-Sequence)1"/1
  connections:
  Three-Phase V-I Measurement25/LConn1 -- Connection Port/RConn1 -- Three-Phase V-I Measurement1/LConn1
  Connection Port1/RConn1 -- Three-Phase V-I Measurement1/LConn2 -- Three-Phase V-I Measurement25/LConn2
  Connection Port2/RConn1 -- Three-Phase V-I Measurement25/LConn3 -- Three-Phase V-I Measurement1/LConn3
  Connection Port3/RConn1 -- Three-Phase V-I Measurement25/RConn1
  Three-Phase V-I Measurement25/RConn2 -- Connection Port4/RConn1
  Three-Phase V-I Measurement25/RConn3 -- Connection Port5/RConn1

== system Y_Model_20_Loads/PMU 4 ==
  "PMU (PLL-Based, Positive-Sequence)1" : powerlib_meascontrol/Measurements/PMU (PLL-Based, Positive-Sequence)  nominalFrequency=50  samplingRate=64  reportingFactor=64
      settings: SourceProductName=Simscape Electrical  SourceProductBaseCode=PS
  "PMU (PLL-Based, Positive-Sequence)2" : powerlib_meascontrol/Measurements/PMU (PLL-Based, Positive-Sequence)  nominalFrequency=50  samplingRate=64  reportingFactor=64
      settings: SourceProductName=Simscape Electrical  SourceProductBaseCode=PS
  Three-Phase V-I Measurement1 : powerlib/Measurements/Three-Phase V-I Measurement  VoltageMeasurement=phase-to-ground  SetLabelV=off  LabelV=Vabc  Vpu=off  VpuLL=off  CurrentMeasurement=no  SetLabelI=off  LabelI=Iabc  Ipu=off  Pbase=100e6  Vbase=500e3  OutputType=Complex  PhasorSimulation=off  PSBequivalent=0
      settings: SourceProductName=Simscape Electrical
  Three-Phase V-I Measurement25 : powerlib/Measurements/Three-Phase V-I Measurement  VoltageMeasurement=no  SetLabelV=off  LabelV=Vabc  Vpu=off  VpuLL=off  CurrentMeasurement=yes  SetLabelI=off  LabelI=Iabc  Ipu=off  Pbase=100e6  Vbase=500e3  OutputType=Complex  PhasorSimulation=off  PSBequivalent=0
      settings: SourceProductName=Simscape Electrical
  To Workspace1 : ToWorkspace  VariableName=i_mag4  SampleTime=-1
  To Workspace2 : ToWorkspace  VariableName=i_ang4  SampleTime=-1
  To Workspace3 : ToWorkspace  VariableName=v_mag4  SampleTime=-1
  To Workspace4 : ToWorkspace  VariableName=v_ang4  SampleTime=-1
  To Workspace5 : ToWorkspace  VariableName=v_freq4  SampleTime=-1
  To Workspace6 : ToWorkspace  VariableName=i_freq4  SampleTime=-1
  Connection Port : PMIOPort  Tag=PMCPort  Side=Left
  Connection Port1 : PMIOPort  Tag=PMCPort  Port=2  Side=Left
  Connection Port2 : PMIOPort  Tag=PMCPort  Port=3  Side=Left
  Connection Port3 : PMIOPort  Tag=PMCPort  Port=4  Side=Right
  Connection Port4 : PMIOPort  Tag=PMCPort  Port=5  Side=Right
  Connection Port5 : PMIOPort  Tag=PMCPort  Port=6  Side=Right
  wires:
  "PMU (PLL-Based, Positive-Sequence)1"/3 -> To Workspace5/1
  "PMU (PLL-Based, Positive-Sequence)1"/2 -> To Workspace4/1
  "PMU (PLL-Based, Positive-Sequence)1"/1 -> To Workspace3/1
  "PMU (PLL-Based, Positive-Sequence)2"/3 -> To Workspace6/1
  "PMU (PLL-Based, Positive-Sequence)2"/1 -> To Workspace1/1
  "PMU (PLL-Based, Positive-Sequence)2"/2 -> To Workspace2/1
  Three-Phase V-I Measurement25/1 -> "PMU (PLL-Based, Positive-Sequence)2"/1
  Three-Phase V-I Measurement1/1 -> "PMU (PLL-Based, Positive-Sequence)1"/1
  connections:
  Three-Phase V-I Measurement25/LConn1 -- Connection Port/RConn1 -- Three-Phase V-I Measurement1/LConn1
  Connection Port1/RConn1 -- Three-Phase V-I Measurement1/LConn2 -- Three-Phase V-I Measurement25/LConn2
  Connection Port2/RConn1 -- Three-Phase V-I Measurement25/LConn3 -- Three-Phase V-I Measurement1/LConn3
  Connection Port3/RConn1 -- Three-Phase V-I Measurement25/RConn1
  Three-Phase V-I Measurement25/RConn2 -- Connection Port4/RConn1
  Three-Phase V-I Measurement25/RConn3 -- Connection Port5/RConn1

== system Y_Model_20_Loads/PMU 5 ==
  "PMU (PLL-Based, Positive-Sequence)1" : powerlib_meascontrol/Measurements/PMU (PLL-Based, Positive-Sequence)  nominalFrequency=50  samplingRate=64  reportingFactor=64
      settings: SourceProductName=Simscape Electrical  SourceProductBaseCode=PS
  "PMU (PLL-Based, Positive-Sequence)2" : powerlib_meascontrol/Measurements/PMU (PLL-Based, Positive-Sequence)  nominalFrequency=50  samplingRate=64  reportingFactor=64
      settings: SourceProductName=Simscape Electrical  SourceProductBaseCode=PS
  Three-Phase V-I Measurement1 : powerlib/Measurements/Three-Phase V-I Measurement  VoltageMeasurement=phase-to-ground  SetLabelV=off  LabelV=Vabc  Vpu=off  VpuLL=off  CurrentMeasurement=no  SetLabelI=off  LabelI=Iabc  Ipu=off  Pbase=100e6  Vbase=500e3  OutputType=Complex  PhasorSimulation=off  PSBequivalent=0
      settings: SourceProductName=Simscape Electrical
  Three-Phase V-I Measurement25 : powerlib/Measurements/Three-Phase V-I Measurement  VoltageMeasurement=no  SetLabelV=off  LabelV=Vabc  Vpu=off  VpuLL=off  CurrentMeasurement=yes  SetLabelI=off  LabelI=Iabc  Ipu=off  Pbase=100e6  Vbase=500e3  OutputType=Complex  PhasorSimulation=off  PSBequivalent=0
      settings: SourceProductName=Simscape Electrical
  To Workspace1 : ToWorkspace  VariableName=i_mag5  SampleTime=-1
  To Workspace2 : ToWorkspace  VariableName=i_ang5  SampleTime=-1
  To Workspace3 : ToWorkspace  VariableName=v_mag5  SampleTime=-1
  To Workspace4 : ToWorkspace  VariableName=v_ang5  SampleTime=-1
  To Workspace5 : ToWorkspace  VariableName=v_freq5  SampleTime=-1
  To Workspace6 : ToWorkspace  VariableName=i_freq5  SampleTime=-1
  Connection Port : PMIOPort  Tag=PMCPort  Side=Left
  Connection Port1 : PMIOPort  Tag=PMCPort  Port=2  Side=Left
  Connection Port2 : PMIOPort  Tag=PMCPort  Port=3  Side=Left
  Connection Port3 : PMIOPort  Tag=PMCPort  Port=4  Side=Right
  Connection Port4 : PMIOPort  Tag=PMCPort  Port=5  Side=Right
  Connection Port5 : PMIOPort  Tag=PMCPort  Port=6  Side=Right
  wires:
  "PMU (PLL-Based, Positive-Sequence)1"/3 -> To Workspace5/1
  "PMU (PLL-Based, Positive-Sequence)1"/2 -> To Workspace4/1
  "PMU (PLL-Based, Positive-Sequence)1"/1 -> To Workspace3/1
  "PMU (PLL-Based, Positive-Sequence)2"/3 -> To Workspace6/1
  "PMU (PLL-Based, Positive-Sequence)2"/1 -> To Workspace1/1
  "PMU (PLL-Based, Positive-Sequence)2"/2 -> To Workspace2/1
  Three-Phase V-I Measurement25/1 -> "PMU (PLL-Based, Positive-Sequence)2"/1
  Three-Phase V-I Measurement1/1 -> "PMU (PLL-Based, Positive-Sequence)1"/1
  connections:
  Three-Phase V-I Measurement25/LConn1 -- Connection Port/RConn1 -- Three-Phase V-I Measurement1/LConn1
  Connection Port1/RConn1 -- Three-Phase V-I Measurement1/LConn2 -- Three-Phase V-I Measurement25/LConn2
  Connection Port2/RConn1 -- Three-Phase V-I Measurement25/LConn3 -- Three-Phase V-I Measurement1/LConn3
  Connection Port3/RConn1 -- Three-Phase V-I Measurement25/RConn1
  Three-Phase V-I Measurement25/RConn2 -- Connection Port4/RConn1
  Three-Phase V-I Measurement25/RConn3 -- Connection Port5/RConn1

== system Y_Model_20_Loads/PMU 6 ==
  "PMU (PLL-Based, Positive-Sequence)1" : powerlib_meascontrol/Measurements/PMU (PLL-Based, Positive-Sequence)  nominalFrequency=50  samplingRate=64  reportingFactor=64
      settings: SourceProductName=Simscape Electrical  SourceProductBaseCode=PS
  "PMU (PLL-Based, Positive-Sequence)2" : powerlib_meascontrol/Measurements/PMU (PLL-Based, Positive-Sequence)  nominalFrequency=50  samplingRate=64  reportingFactor=64
      settings: SourceProductName=Simscape Electrical  SourceProductBaseCode=PS
  Three-Phase V-I Measurement1 : powerlib/Measurements/Three-Phase V-I Measurement  VoltageMeasurement=phase-to-ground  SetLabelV=off  LabelV=Vabc  Vpu=off  VpuLL=off  CurrentMeasurement=no  SetLabelI=off  LabelI=Iabc  Ipu=off  Pbase=100e6  Vbase=500e3  OutputType=Complex  PhasorSimulation=off  PSBequivalent=0
      settings: SourceProductName=Simscape Electrical
  Three-Phase V-I Measurement25 : powerlib/Measurements/Three-Phase V-I Measurement  VoltageMeasurement=no  SetLabelV=off  LabelV=Vabc  Vpu=off  VpuLL=off  CurrentMeasurement=yes  SetLabelI=off  LabelI=Iabc  Ipu=off  Pbase=100e6  Vbase=500e3  OutputType=Complex  PhasorSimulation=off  PSBequivalent=0
      settings: SourceProductName=Simscape Electrical
  To Workspace1 : ToWorkspace  VariableName=i_mag6  SampleTime=-1
  To Workspace2 : ToWorkspace  VariableName=i_ang6  SampleTime=-1
  To Workspace3 : ToWorkspace  VariableName=v_mag6  SampleTime=-1
  To Workspace4 : ToWorkspace  VariableName=v_ang6  SampleTime=-1
  To Workspace5 : ToWorkspace  VariableName=v_freq6  SampleTime=-1
  To Workspace6 : ToWorkspace  VariableName=i_freq6  SampleTime=-1
  Connection Port : PMIOPort  Tag=PMCPort  Side=Left
  Connection Port1 : PMIOPort  Tag=PMCPort  Port=2  Side=Left
  Connection Port2 : PMIOPort  Tag=PMCPort  Port=3  Side=Left
  Connection Port3 : PMIOPort  Tag=PMCPort  Port=4  Side=Right
  Connection Port4 : PMIOPort  Tag=PMCPort  Port=5  Side=Right
  Connection Port5 : PMIOPort  Tag=PMCPort  Port=6  Side=Right
  wires:
  "PMU (PLL-Based, Positive-Sequence)1"/3 -> To Workspace5/1
  "PMU (PLL-Based, Positive-Sequence)1"/2 -> To Workspace4/1
  "PMU (PLL-Based, Positive-Sequence)1"/1 -> To Workspace3/1
  "PMU (PLL-Based, Positive-Sequence)2"/3 -> To Workspace6/1
  "PMU (PLL-Based, Positive-Sequence)2"/1 -> To Workspace1/1
  "PMU (PLL-Based, Positive-Sequence)2"/2 -> To Workspace2/1
  Three-Phase V-I Measurement25/1 -> "PMU (PLL-Based, Positive-Sequence)2"/1
  Three-Phase V-I Measurement1/1 -> "PMU (PLL-Based, Positive-Sequence)1"/1
  connections:
  Three-Phase V-I Measurement25/LConn1 -- Connection Port/RConn1 -- Three-Phase V-I Measurement1/LConn1
  Connection Port1/RConn1 -- Three-Phase V-I Measurement1/LConn2 -- Three-Phase V-I Measurement25/LConn2
  Connection Port2/RConn1 -- Three-Phase V-I Measurement25/LConn3 -- Three-Phase V-I Measurement1/LConn3
  Connection Port3/RConn1 -- Three-Phase V-I Measurement25/RConn1
  Three-Phase V-I Measurement25/RConn2 -- Connection Port4/RConn1
  Three-Phase V-I Measurement25/RConn3 -- Connection Port5/RConn1
